simulink model "simulink_model"  (R2024b)
settings: Solver=FixedStepDiscrete  StartTime=0.0  StopTime=10.0  FixedStep=0.1  RelTol=1e-3  EnableMultiTasking=on
libraries: stm32f4xxblockslib x8, stm32blockslib x2
settings Model: STM32="{\"DigitalPortWrite\":[{\"ID\":\"untitled:4\"},{\"ID\":\"progetto:4\"},{\"ID\":\"progetto_gruppo17:4\"},{\"ID\":\"progetto_gruppo17:23\"},{\"ID\":\"progetto_gruppo17_05_06_2025:23\"},{\"ID\":\"progetto_gruppo17_05_06_2025:4\"},{\"ID\":\"progetto_gruppo17_06_06_2025:23\"},{\"ID\":\"progetto_gruppo17_06_06_2025:4\"},{\"ID\":\"progetto_gruppo17_06_06_2025_vers_a:4\"},{\"ID\":\"progetto_gruppo17_06_06_2025_vers_a:23\"},{\"ID\":\"progetto_se_gruppo_17:23\"},{\"ID\":\"progetto_se_gruppo_17:4\"}],\"DigitalPortRead\":[{\"ID\":\"untitled:5\"},{\"ID\":\"progetto:5\"},{\"ID\":\"progetto_gruppo17:5\"},{\"ID\":\"progetto_gruppo17:22\"},{\"ID\":\"progetto_gruppo17:24\"},{\"ID\":\"progetto_gruppo17:29\"},{\"ID\":\"progetto_gruppo17_05_06_2025:29\"},{\"ID\":\"progetto_gruppo17_05_06_2025:24\"},{\"ID\":\"progetto_gruppo17_05_06_2025:22\"},{\"ID\":\"progetto_gruppo17_05_06_2025:5\"},{\"ID\":\"progetto_gruppo17_06_06_2025:29\"},{\"ID\":\"progetto_gruppo17_06_06_2025:24\"},{\"ID\":\"progetto_gruppo17_06_06_2025:22\"},{\"ID\":\"progetto_gruppo17_06_06_2025:5\"},{\"ID\":\"progetto_gruppo17_06_06_2025_vers_a:5\"},{\"ID\":\"progetto_gruppo17_06_06_2025_vers_a:22\"},{\"ID\":\"progetto_gruppo17_06_06_2025_vers_a:24\"},{\"ID\":\"progetto_gruppo17_06_06_2025_vers_a:29\"},{\"ID\":\"progetto_se_gruppo_17:29\"},{\"ID\":\"progetto_se_gruppo_17:24\"},{\"ID\":\"progetto_se_gruppo_17:22\"},{\"ID\":\"progetto_se_gruppo_17:5\"}],\"UARTWrite\":[{\"ID\":\"untitled:10\"},{\"ID\":\"progetto:10\"},{\"ID\":\"progetto_gruppo17:10\"},{\"ID\":\"progetto_gruppo17_05_06_2025:10\"},{\"ID\":\"progetto_gruppo17_06_06_2025:10\"},{\"ID\":\"progetto_gruppo17_06_06_2025_vers_a:10\"},{\"ID\":\"progetto_se_gruppo_17:10\"}],\"UARTRead\":[{\"ID\":\"untitled:20\"},{\"ID\":\"progetto:20\"},{\"ID\":\"progetto_gruppo17:20\"},{\"ID\":\"progetto_gruppo17_05_06_2025:20\"},{\"ID\":\"progetto_gruppo17_06_06_2025:20\"},{\"ID\":\"progetto_gruppo17_06_06_2025_vers_a:20\"},{\"ID\":\"progetto_se_gruppo_17:20\"}],\"PWMOutput\":[{\"ID\":\"progetto_gruppo17:26\"},{\"ID\":\"progetto_gruppo17_05_06_2025:26\"},{\"ID\":\"progetto_gruppo17_05_06_2025:30\"},{\"ID\":\"progetto_gruppo17_06_06_2025:26\"},{\"ID\":\"progetto_gruppo17_06_06_2025:30\"},{\"ID\":\"progetto_gruppo17_06_06_2025_vers_a:30\"},{\"ID\":\"progetto_gruppo17_06_06_2025_vers_a:26\"},{\"ID\":\"progetto_se_gruppo_17:26\"},{\"ID\":\"progetto_se_gruppo_17:30\"}]}"  Creator=simon  LastModifiedBy=simon
settings OptimizationCC: DefaultParameterBehavior=Inlined  EnhancedBackFolding=on  PassReuseOutputArgsAs=Individual arguments  ZeroExternalMemoryAtStartup=off  ZeroInternalMemoryAtStartup=off  MaxStackSize=512  OptimizeBlockOrder=speed  DifferentSizesBufferReuse=on  OptimizationCustomize=off  EfficientTunableParamExpr=on
settings DebuggingCC: ParameterTunabilityLossMsg=error
settings HardwareCC: ProdBitPerPointer=32  ProdBitPerSizeT=32  ProdBitPerPtrDiffT=32  ProdLargestAtomicInteger=Long  ProdLargestAtomicFloat=Double  ProdWordSize=32  ProdLongLongMode=on  ProdHWDeviceType=ARM Compatible->ARM Cortex-M
settings SFSimCC: MATLABDynamicMemAlloc=off
settings RTWCC: Description=Embedded Coder  SystemTargetFile=ert.tlc  HardwareBoard=STM32G4xx Based  TemplateMakefile=ert_default_tmf  Toolchain=GNU Tools for ARM Embedded Processors
settings CodeAppCC: ForceParamTrailComments=on  IgnoreCustomStorageClasses=off  OperatorAnnotations=on  SimulinkDataObjDesc=on  SFDataObjDesc=on  InsertBlockDesc=on
settings ERTTargetCC: TargetLangStandard=C99 (ISO)  CodeReplacementLibrary=ARM Cortex-M  SupportVariableSizeSignals=on  ExtModeTransport=3  ExtModeStaticAlloc=on  ExtModeStaticAllocSize=2048  ExtModeMexFile=ext_xcp  ExtModeIntrfLevel=Level2 - Open  DynamicArrayContainerType=coder::array

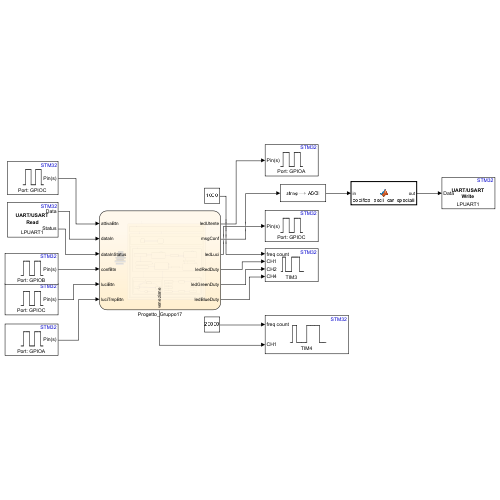
[thumbnail: Simulink's stored preview of the top-level diagram]
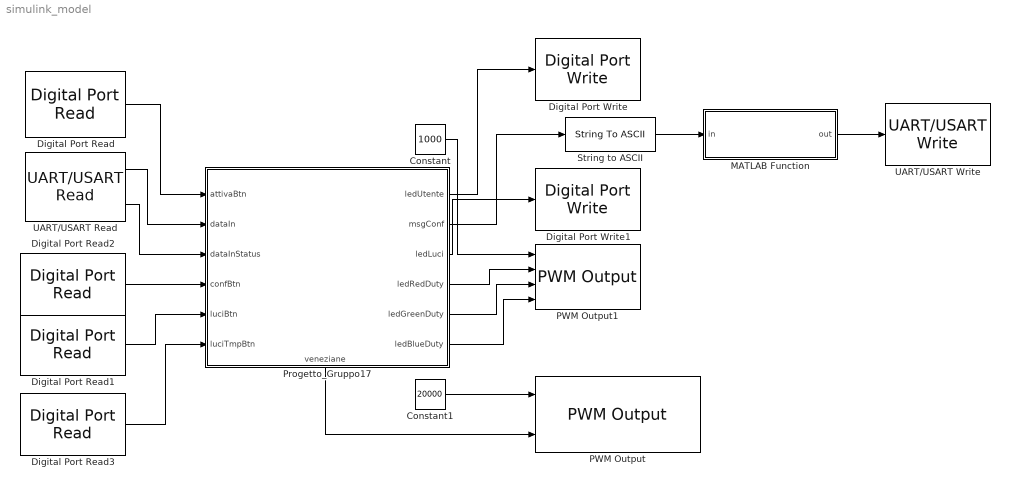
== system simulink_model ==
  Constant : Constant  Value=1000
  Constant1 : Constant  Value=20000
  Digital Port Read : stm32f4xxblockslib/Digital Port Read  PortName=GPIOC  PinNumber=[13]  ReadOperation=on  IOAsArray=on  SampleTime=-1  EnableSimPort=off  hoistedMaskSrc=ECSoC/ECSimCodegen/Digital Port Read
      settings: LibrarySourceBlock=stm32f2xxblockslib/Digital Port Read
  Digital Port Read1 : stm32f4xxblockslib/Digital Port Read  PortName=GPIOC  PinNumber=[10]  ReadOperation=on  IOAsArray=on  SampleTime=-1  EnableSimPort=off  hoistedMaskSrc=ECSoC/ECSimCodegen/Digital Port Read
      settings: LibrarySourceBlock=stm32f3xxblockslib/Digital Port Read
  Digital Port Read2 : stm32f4xxblockslib/Digital Port Read  PortName=GPIOB  PinNumber=[0]  ReadOperation=on  IOAsArray=on  SampleTime=-1  EnableSimPort=off  hoistedMaskSrc=ECSoC/ECSimCodegen/Digital Port Read
      settings: LibrarySourceBlock=stm32f3xxblockslib/Digital Port Read
  Digital Port Read3 : stm32f4xxblockslib/Digital Port Read  PortName=GPIOA  PinNumber=[15]  ReadOperation=on  IOAsArray=on  SampleTime=-1  EnableSimPort=off  hoistedMaskSrc=ECSoC/ECSimCodegen/Digital Port Read
      settings: LibrarySourceBlock=stm32f3xxblockslib/Digital Port Read
  Digital Port Write : stm32f4xxblockslib/Digital Port Write  PortName=GPIOA  PinNumber=[5]  ReadOperation=off  IOAsArray=on  EnableSimPort=off  hoistedMaskSrc=ECSoC/ECSimCodegen/Digital Port Write
      settings: LibrarySourceBlock=stm32f3xxblockslib/Digital Port Write
  Digital Port Write1 : stm32f4xxblockslib/Digital Port Write  PortName=GPIOC  PinNumber=[2]  ReadOperation=off  IOAsArray=on  EnableSimPort=off  hoistedMaskSrc=ECSoC/ECSimCodegen/Digital Port Write
      settings: LibrarySourceBlock=stm32f3xxblockslib/Digital Port Write
  MATLAB Function : MATLAB Function  TreatAsAtomicUnit=on
  PWM Output : stm32f4xxblockslib/PWM Output  TimerModule=TIM4  DutycycleUnits=Counts  EnableChannel1=on  EnableChannel2=off  EnableChannel3=off  EnableChannel4=off  EnableCounterInput=off  EnableMainOutputInput=off  EnableFrequencyInput=on  SetRCAfterCE=off  OutputDirection=off  OutputMainOutputEnableStatus=off  SampleTime=0.1  EnableSimPort=off  EnableUpdateEvent=off  EnableCaptureCompare1Event=off  EnableCaptureCompare2Event=off  EnableCaptureCompare3Event=off  EnableCaptureCompare4Event=off  EnableTriggerEvent=off  EnableBreakEvent=off  ProcessorFamily=STM32F4  hoistedMaskSrc=ECSoC/ECSimCodegen/PWM Output
      settings: LibrarySourceBlock=stm32f2xxblockslib/PWM Output
  PWM Output1 : stm32f4xxblockslib/PWM Output  TimerModule=TIM3  DutycycleUnits=Percentage  EnableChannel1=on  EnableChannel2=on  EnableChannel3=off  EnableChannel4=on  EnableCounterInput=off  EnableMainOutputInput=off  EnableFrequencyInput=on  SetRCAfterCE=off  OutputDirection=off  OutputMainOutputEnableStatus=off  SampleTime=0.1  EnableSimPort=off  EnableUpdateEvent=off  EnableCaptureCompare1Event=off  EnableCaptureCompare2Event=off  EnableCaptureCompare3Event=off  EnableCaptureCompare4Event=off  EnableTriggerEvent=off  EnableBreakEvent=off  ProcessorFamily=STM32F3  hoistedMaskSrc=ECSoC/ECSimCodegen/PWM Output
      settings: LibrarySourceBlock=stm32f3xxblockslib/PWM Output
  Progetto_Gruppo17 : Stateflow chart  TreatAsAtomicUnit=on
      settings: PortSchema="{\"entries\":[{\"content\":{\"sides\":[{\"content\":{\"connectorIds\":[\"In1\",\"In2\",\"In3\",\"In4\",\"In5\",\"In6\"]},\"type\":\"ConnectorPlacement.EquallySpacedRectSide\",\"uuid\":\"75f39260-4103-4749-81bf-ba76d3f8645b\"},{\"content\":{\"connectorIds\":[\"Out2\",\"Out3\",\"Out4\",\"Out7\",\"Out6\",\"Out5\"],\"side\":\"RIGHT\"},\"type\":\"ConnectorPlacement.EquallySpacedRectSide\",\"uuid\":\"22f09110-723e-4154-922d-9361e0bfb65a\"},{\"content\":{\"side\":\"TOP\"},\"type\":\"ConnectorPlacement.EquallySpacedRectSide\",\"uuid\":\"fa7b379e-0fd5-4b5f-9158-63c7f34f09a8\"},{\"content\":{\"connectorIds\":[\"Out1\"],\"side\":\"BOTTOM\"},\"type\":\"ConnectorPlacement.EquallySpacedRectSide\",\"uuid\":\"f8770b9f-bc27-4bf9-8903-206540cbe1f9\"}]},\"type\":\"ConnectorPlacement.EquallySpacedConnector\",\"uuid\":\"436e63a6-7db2-4b6a-ab66-b755d4d8d881\"}],\"packageUris\":[\"http://schema.mathworks.com/mf0/Connector/R2020b\"],\"version\":\"1.0\"}"
  String to ASCII : StringToASCII  OutputVectorSize=100
  UART/USART Read : stm32blockslib/UART//USART Read  UARTModule=LPUART1  DataType=uint8  DataLength=1  BlockingMode=off  BlockingTimeout=0.1  OutputLength=off  OutputStatus=on  SampleTime=-1
      settings: LibrarySourceBlock=stm32f2xxblockslib/UART//USART Read
  UART/USART Write : stm32blockslib/UART//USART Write  UARTModule=LPUART1  LengthOfDataToSend=off  BlockingMode=off  BlockingTimeout=0.1  OutputStatus=off
      settings: LibrarySourceBlock=stm32g4xxblockslib/UART//USART Write
  wires:
  Digital Port Read1/1 -> Progetto_Gruppo17/5(luciBtn)
  Digital Port Read3/1 -> Progetto_Gruppo17/6(luciTmpBtn)
  Constant/1 -> PWM Output1/1
  Digital Port Read/1 -> Progetto_Gruppo17/1(attivaBtn)
  Digital Port Read2/1 -> Progetto_Gruppo17/4(confBtn)
  UART/USART Read/2 -> Progetto_Gruppo17/3(dataInStatus)
  UART/USART Read/1 -> Progetto_Gruppo17/2(dataIn)
  Progetto_Gruppo17/1(veneziane) -> PWM Output/2
  Progetto_Gruppo17/6(ledGreenDuty) -> PWM Output1/3
  Progetto_Gruppo17/2(ledUtente) -> Digital Port Write/1
  Progetto_Gruppo17/7(ledRedDuty) -> PWM Output1/2
  Progetto_Gruppo17/3(msgConf) -> String to ASCII/1
  Progetto_Gruppo17/4(ledLuci) -> Digital Port Write1/1
  Progetto_Gruppo17/5(ledBlueDuty) -> PWM Output1/4
  Constant1/1 -> PWM Output/1
  String to ASCII/1 -> MATLAB Function/1(in)
  MATLAB Function/1(out) -> UART/USART Write/1

== stateflow chart simulink_model/Progetto_Gruppo17 ==
  state SistemaDomotica
    state SistemaInattivo
      en:attiva_btn_prev = attivaBtn;
      msgConf = "\033[0;0H\033[2JDISPOSITIVO INATTIVO :("
      ledUtente = OFF;
      ledLuci = OFF;
      ledBlueDuty = 100;
      ledGreenDuty = 0;
      ledRedDuty = 0;
      veneziane = dutyVeneziane(0);
      du: attiva_btn_prev = attivaBtn;
      msgConf = "";
    state SistemaAttivo
      en: attiva_btn_prev = attivaBtn;
      du: attiva_btn_prev = attivaBtn;
      state LedToggle [parallel]
        settings: executionOrder=1
        state LedOff
          en: ledUtente=OFF;
        state LedOn
          en: ledUtente=ON;
        (default) -> LedOn
        LedOn -> LedOff : after(0.5,sec)
        LedOff -> LedOn : after(0.5,sec)
      state ModSistema [parallel]
        settings: executionOrder=2
        state ConfigurazioneDispositivo
          en: conf_btn_prev = confBtn;
          du: conf_btn_prev = confBtn;
          state RicezioneStatoLuci
            en: valid=2; stato_luci = 2;
            if dataIn == char(13)
            [valid,stato_luci] = verificaValoreLuci(buffer);
            if stato_luci == TRUE && valid == TRUE
            msgConf = " -> ACCESE\n\r";
            elseif stato_luci == FALSE && valid == TRUE
            msgConf = " -> SPENTE\n\r";
            elseif valid == FALSE
            msgConf = "-> ERRORE\033[2K\r";
            end
            else
            [buffer, buffer_index, message] = gestisciBufferInput(dataIn, buffer, buffer_index,2);
            msgConf = string(char(message));
            end
            du:  msgConf = "";
          state RicezioneConfVeneziane
            en: valid = 2;
            if dataIn == char(13)
            gradi_veneziana_in = conversioneNum(buffer,buffer_index);
            valid = verificaValoreVeneziane(gradi_veneziana_in);
            if valid == TRUE
            msgConf = " -> OK\n\r";
            else
            msgConf = "-> ERRORE\033[2K\r";
            end
            buffer_index = 1;
            else
            [buffer, buffer_index, message] = gestisciBufferInput(dataIn, buffer, buffer_index,4);
            msgConf = string(char(message));
            end
            du:  msgConf = "";
          state StampaConfVeneziane
            en: msgConf="Configura veneziane - [0:180] (Gradi) - Risoluzione [20] (Gradi): ";
            buffer_index=1;
            du: msgConf="";
          state StampaConfStatoLuce
            en: msgConf="Configura luci - [a/A (Accese), s/S (Spente)]: ";
            buffer_index=1;
            du: msgConf="";
          state StampaConfTempLuce
            en: msgConf="Inserisci un valore di temporizzazione - [0] (Inattiva) - [5:30] (Secondi): ";
            buffer_index=1;
            du: msgConf="";
          state InizioConfigurazione
            en: conf_setted = FALSE;
            if valid_conf == TRUE
            msgConf = "\033[0;0H\033[2JMOD CONF [::]\n\r[EXIT MODE] Premi CONF_BTN per uscire...\n\r";
            else
            msgConf = "\033[0;0H\033[2JMOD CONF [::]\n\r";
            end
          state RicezioneTemperatura
            en: valid=2;
            if dataIn == char(13)
            temperatura = conversioneNum(buffer,buffer_index);
            valid = conversioneValoreTemperatura(temperatura);
            if valid == TRUE
            msgConf = " -> OK\n\r";
            else
            msgConf = "->ERRORE\033[2K\r";
            end
            buffer_index = 1;
            else
            [buffer, buffer_index, message] = gestisciBufferInput(dataIn, buffer, buffer_index,3);
            msgConf = string(char(message));
            end
            du:  msgConf = "";
          state RicezioneTempLuci
            en: valid=2;
            if dataIn == char(13)
            temporizzazione = conversioneNum(buffer,buffer_index);
            valid = conversioneValoreTemporizzazione(temporizzazione);
            if valid == TRUE
            msgConf = " -> OK\n\r";
            else
            msgConf = "-> ERRORE\033[2K\r";
            end
            buffer_index = 1;
            else
            [buffer, buffer_index, message] = gestisciBufferInput(dataIn, buffer, buffer_index,3);
            msgConf = string(char(message));
            end
            du:  msgConf = "";
          state FineConfigurazione
            en: conf_setted = TRUE; msgConf = "CONF DONE -> CONF EXIT\n"; valid_conf = TRUE;
            veneziane_conf_val = gradi_veneziana_in;
            stato_luci_conf_val = stato_luci;
            temp_luci_conf_val = temporizzazione;
            temperatura_conf_val = temperatura;
          state StampaConfTemperatura
            en: msgConf="Configura temperatura - [16:30] (Gradi): ";
            buffer_index=1;
            du: msgConf="";
          RicezioneStatoLuci -> RicezioneStatoLuci [order 1] : [dataInStatus==0]
          RicezioneConfVeneziane -> RicezioneConfVeneziane [order 1] : [dataInStatus==0]
          StampaConfVeneziane -> RicezioneConfVeneziane : [dataInStatus==0]
          StampaConfStatoLuce -> RicezioneStatoLuci : [dataInStatus==0]
          RicezioneConfVeneziane -> StampaConfStatoLuce [order 3] : [valid==TRUE]
          RicezioneConfVeneziane -> StampaConfVeneziane [order 2] : [valid==FALSE]
          RicezioneStatoLuci -> StampaConfStatoLuce [order 2] : [valid == FALSE]
          InizioConfigurazione -> StampaConfVeneziane : [conf_setted==FALSE]
          RicezioneStatoLuci -> StampaConfTempLuce [order 3] : [valid == TRUE]
          StampaConfTempLuce -> RicezioneTempLuci : [dataInStatus == 0]
          RicezioneTempLuci -> StampaConfTempLuce [order 2] : [valid == FALSE]
          RicezioneTempLuci -> RicezioneTempLuci [order 3] : [dataInStatus == 0]
          (default) -> InizioConfigurazione
          RicezioneTemperatura -> RicezioneTemperatura [order 2] : [dataInStatus == 0]
          RicezioneTemperatura -> FineConfigurazione [order 3] : [valid == TRUE]
          StampaConfTemperatura -> RicezioneTemperatura : [dataInStatus == 0]
          RicezioneTempLuci -> StampaConfTemperatura [order 1] : [valid == TRUE]
          RicezioneTemperatura -> StampaConfTemperatura [order 1] : [valid == FALSE]
        state EsecuzioneDispositivo
          en: conf_btn_prev = confBtn;
          msgConf = "\033[0;0H\033[2J";
          du: conf_btn_prev = confBtn;
          state StampaStato [parallel]
            settings: executionOrder=4
            state StatoVenezianeValue
              en: msgConf =string(veneziane_conf_val);
              du: msgConf = "";
            state StatoLuci
              if ledLuci == OFF
              msgConf = " gradi\n\rLuci: spente";
              else
              msgConf = " gradi\n\rLuci: accese";
              end
              du: msgConf = "";
            state StatoLuciTemporizzateDialog
              en: msgConf="\n\rDurata temporizzazione: "
              du: msgConf="";
            state StatoVenezianeDialog
              en: msgConf = "Veneziane: ";
              du: msgConf = "";
            state StatoLuciTemporizzateValue
              en: msgConf = string(temp_luci_conf_val);
              du: msgConf = "";
            state StatoOperativo
              msgConf = "\033[0;0H\033[2JMOD OPERATIVA ::>\n\r";
              du: msgConf = "";
            state StatoTemperaturaDialog
              en: msgConf = " sec\n\rTemperatura: ";
              du: msgConf= "";
            state StatoTemperaturaValue
              en: msgConf = string(temperatura_conf_val);
              du: msgConf= "";
            state StatoTemperaturaValue1
              en: msgConf = " gradi";
              du: msgConf= "";
            StatoVenezianeValue -> StatoLuci : [1]
            StatoLuci -> StatoLuciTemporizzateDialog : [1]
            StatoVenezianeDialog -> StatoVenezianeValue : [1]
            StatoLuciTemporizzateDialog -> StatoLuciTemporizzateValue : [1]
            StatoOperativo -> StatoVenezianeDialog : [1]
            (default) -> StatoOperativo
            StatoLuciTemporizzateValue -> StatoTemperaturaDialog : [1]
            StatoTemperaturaValue1 -> StatoOperativo : [after(10,sec)]
            StatoTemperaturaDialog -> StatoTemperaturaValue : [1]
            StatoTemperaturaValue -> StatoTemperaturaValue1 : [1]
          state GestoreTemperatura [parallel]
            en: [ledRedDuty, ledGreenDuty, ledBlueDuty]=cambioDuty(temperatura_conf_val);
            settings: executionOrder=1
          state GestoreVeneziane [parallel]
            en: veneziane = dutyVeneziane(veneziane_conf_val);
            settings: executionOrder=3
          state GestoreLuci [parallel]
            settings: executionOrder=2
            state AcceseTemp
              en:ledLuci = ON;
              luci_btn_prev = luciBtn;
              du: luci_btn_prev = luciBtn;
            state Spente
              en: ledLuci = OFF;
              luci_btn_prev = luciBtn;
              luci_temp_btn_prev = luciTmpBtn;
              du: luci_btn_prev = luciBtn;
              luci_temp_btn_prev = luciTmpBtn;
            state Accese
              en: ledLuci = ON;
              luci_btn_prev = luciBtn;
              luci_temp_btn_prev = luciTmpBtn;
              du: luci_btn_prev = luciBtn;
              luci_temp_btn_prev = luciTmpBtn;
            state StatoIniziale
              en: ledLuci = OFF;
            Spente -> AcceseTemp [order 2] : [temp_luci_conf_val ~= 0 && luci_temp_btn_prev == PRESSED && luciTmpBtn == NOTPRESSED]{luci_temp_btn_prev = luciTmpBtn;}
            Accese -> AcceseTemp [order 2] : [temp_luci_conf_val ~= 0 && luci_temp_btn_prev == PRESSED && luciTmpBtn == NOTPRESSED]{luci_temp_btn_prev = luciTmpBtn;}
            AcceseTemp -> Spente : [after(temp_luci_conf_val,sec) || (luci_btn_prev == PRESSED && luciBtn == NOTPRESSED)]{luci_btn_prev = luciBtn;}
            Accese -> Spente [order 1] : [luci_btn_prev == PRESSED && luciBtn == NOTPRESSED]{luci_btn_prev = luciBtn;}
            Spente -> Accese [order 1] : [luci_btn_prev == PRESSED && luciBtn == NOTPRESSED]{luci_btn_prev = luciBtn;}
            StatoIniziale -> Spente [order 1] : [stato_luci_conf_val == OFF]
            StatoIniziale -> Accese [order 2] : [stato_luci_conf_val == ON]
            (default) -> StatoIniziale
        (default) -> ConfigurazioneDispositivo
        ConfigurazioneDispositivo -> EsecuzioneDispositivo : [conf_setted == TRUE || (valid_conf == TRUE && confBtn == NOTPRESSED && conf_btn_prev == PRESSED)]{conf_btn_prev = confBtn;}
        EsecuzioneDispositivo -> ConfigurazioneDispositivo : [confBtn == NOTPRESSED && conf_btn_prev == PRESSED]{conf_btn_prev = confBtn;}
    (default) -> SistemaInattivo
    SistemaInattivo -> SistemaAttivo : [attivaBtn == NOTPRESSED && attiva_btn_prev == PRESSED]{attiva_btn_prev = attivaBtn}
    SistemaAttivo -> SistemaInattivo : [attivaBtn == NOTPRESSED && attiva_btn_prev == PRESSED]{attiva_btn_prev = attivaBtn;}
  (default) -> SistemaDomotica : {
      | attiva_btn_prev = NOTPRESSED;
      | conf_btn_prev = NOTPRESSED;
      | luci_btn_prev = NOTPRESSED;
      | luci_temp_btn_prev = NOTPRESSED;
      | conf_setted = FALSE;
      | }
  data: buff function_input; valido function_output; luci function_output; buff function_input; val function_output; buff_index function_input; valido function_output; gradi function_input; temp function_input; valido function_output; d function_input; buff function_input; buff_index function_input; buff function_output; buff_index function_output; msg function_output uint8; dimensione function_input; temp function_input; valido function_output; duty_red function_output; duty_green function_output; duty_blue function_output; temp function_input; gradi_ven function_input; impulso function_output; veneziane output =1; attivaBtn input; ledUtente output; msgConf output string =""; NOTPRESSED constant boolean =0; OFF constant double =0; ON constant double =1; PRESSED constant boolean =1; dataIn input uint8; dataInStatus input; buffer local uint8 size=6 =zeros(6,1); buffer_index local uint8; gradi_veneziana_in local uint8 =0; valid local uint8; message local uint8; stato_luci local uint8; temporizzazione local uint8; confBtn input; conf_setted local double =0; temperatura local uint8; luciBtn input; ledLuci output; stato_luci_conf_val local uint8 =0; temp_luci_conf_val local uint8 =0; temperatura_conf_val local uint8 =16; veneziane_conf_val local uint8 =0; valid_conf local double =0; ledBlueDuty output uint8 =100; ledGreenDuty output uint8 =0; ledRedDuty output uint8 =0; luciTmpBtn input; FALSE constant double =0; TRUE constant double =1; attiva_btn_prev local; conf_btn_prev local; luci_btn_prev local; luci_temp_btn_prev local
  function [valido,luci] = verificaValoreLuci(buff):
    | function [valido,luci] = verificaValoreLuci(buff)
    |     
    |     if buff(1) == char(65) || buff(1) == char(97)
    |          valido = uint8(1);
    |          luci = uint8(1);
    |     elseif buff(1) == char(83) || buff(1) == char(115)
    |          valido = uint8(1);
    |          luci = uint8(0);
    |     else
    |         valido = uint8(0);
    |         luci = uint8(2);
    |     end
    | 
    | end
  function val = conversioneNum(buff, buff_index):
    | function val = conversioneNum(buff, buff_index)
    | 
    |     val = uint8(0);
    |     j = uint8(1);
    | 
    |     while j < buff_index
    |         c = buff(j);
    |         if c >= uint8(48) && c <= uint8(57)
    |             val = val * uint8(10) + (c - uint8(48));
    |             j = j + 1;
    |         else
    |             val = uint8(255);  
    |             break;
    |         end
    |     end
    | end
  function valido = verificaValoreVeneziane(gradi):
    | function valido = verificaValoreVeneziane(gradi)
    |     if mod(gradi,20) == 0 && gradi >= 0 && gradi <= 180
    |         valido = uint8(1);
    |     else
    |         valido = uint8(0);
    |     end
    | end
  function valido = conversioneValoreTemporizzazione(temp):
    | function valido = conversioneValoreTemporizzazione(temp)
    |     if  temp >= 5 && temp <= 30 || temp == 0
    |         valido = uint8(1);
    |     else
    |         valido = uint8(0);
    |     end
    | end
  function [buff, buff_index,msg] = gestisciBufferInput(d, buff, buff_index,dimensione):
    | function [buff, buff_index,msg] = gestisciBufferInput(d, buff, buff_index,dimensione)
    |     
    |     msg = uint8(0);
    |     if  buff_index < dimensione && d ~= char(127)
    |         % Aggiunta normale di carattere
    |         buff(buff_index) = d;
    |         buff_index = buff_index + 1;
    |         msg = d;
    |     elseif d == char(127) && buff_index > 1
    |         % Backspace
    |         buff_index = buff_index - 1;
    |         msg = d;
    |     end
    | end
  function valido = conversioneValoreTemperatura(temp):
    | function valido = conversioneValoreTemperatura(temp)
    |     if  temp >= 16 && temp <= 30
    |         valido = uint8(1);
    |     else
    |         valido = uint8(0);
    |     end
    | end
  function [duty_red, duty_green, duty_blue] = cambioDuty(temp):
    | function [duty_red, duty_green, duty_blue] = cambioDuty(temp)
    | 
    | %blu
    | if temp >=16 && temp <=18
    |     duty_red = uint8(0);
    |     duty_green = uint8(0);
    |     duty_blue = uint8(100);
    | 
    | %viola
    | elseif temp >=19 && temp <=21
    |     duty_red = uint8(50);
    |     duty_green = uint8(0);
    |     duty_blue = uint8(50);
    | 
    | %giallo
    | elseif temp >= 22 && temp <=24
    |     duty_red = uint8(100);
    |     duty_green = uint8(10);
    |     duty_blue = uint8(0);
    | 
    | %arancione
    | elseif temp >= 25 && temp <= 27
    |     duty_red = uint8(100);
    |     duty_green = uint8(3);
    |     duty_blue = uint8(0);
    | 
    | %rosso
    | else
    |     duty_red = uint8(100);
    |     duty_green = uint8(0);
    |     duty_blue = uint8(0);
    | 
    | end
  function impulso = dutyVeneziane(gradi_ven):
    | function impulso = dutyVeneziane(gradi_ven)
    | 
    | gradi = double(gradi_ven);
    | impulso = 500 + (gradi *(2500 - 500) / 180);
    | 
    | end

== matlab function simulink_model/MATLAB Function ==
  data: in input; out output uint8 size=100
function out = codifica_ascii_car_speciali(in)

% Lunghezza massima supportata (personalizzabile)
MAX_LEN = 100;

% Preallocazione con lunghezza fissa
out = zeros(MAX_LEN,1, 'uint8');
len_out = 0;

i = 1;
while i <= length(in) && len_out < MAX_LEN
    
    if i + 15 <= length(in)
        if in(i)   == 92 && in(i+1) == 48 && in(i+2) == 51 && in(i+3) == 51 && ...
           in(i+4) == 91 && in(i+5) == 48 && in(i+6) == 59 && in(i+7) == 48 && ...
           in(i+8) == 72 && in(i+9) == 92 && in(i+10) == 48 && in(i+11) == 51 && ...
           in(i+12) == 51 && in(i+13) == 91 && in(i+14) == 50 && in(i+15) == 74
       
            if len_out + 10 <= MAX_LEN
                out(len_out+1:len_out+10) = uint8([27 91 48 59 48 72 27 91 50 74]);
                len_out = len_out + 10;
            end
            i = i + 16;
            continue;
        end
    end


    % Riconoscimento \033[2K = [92 48 51 51 91 50 75]
    if i + 6 <= length(in) && ...
       in(i)   == 92  && ...  % '\'
       in(i+1) == 48  && ...  % '0'
       in(i+2) == 51  && ...  % '3'
       in(i+3) == 51  && ...  % '3'
       in(i+4) == 91  && ...  % '['
       in(i+5) == 50  && ...  % '2'
       in(i+6) == 75          % 'K'
   
        % Sostituisci con [27 91 50 75]
        if len_out + 4 <= MAX_LEN
            out(len_out+1:len_out+4) = uint8([27 91 50 75]);
            len_out = len_out + 4;
        end
        i = i + 7;
        continue;
    end

    if in(i) == 92 && i < length(in)  % 92 == backslash '\'
        i = i + 1;
        if i <= length(in)
            c = in(i);
            esc_val = 0;
            switch c
                case 110  % 'n'
                    esc_val = 10;
                case 114  % 'r'
                    esc_val = 13;
                case 116  % 't'
                    esc_val = 9;
                case 92   % '\'
                    esc_val = 92;
                case 39   % '''
                    esc_val = 39;
                case 34   % '"'
                    esc_val = 34;
                otherwise
                    % Non riconosciuto, aggiungi '\' e il carattere successivo
                    len_out = len_out + 1;
                    out(len_out) = uint8(92);
                    if len_out < MAX_LEN
                        len_out = len_out + 1;
                        out(len_out) = uint8(c);
                    end
                    i = i + 1;
                    continue;
            end
            len_out = len_out + 1;
            out(len_out) = uint8(esc_val);
        end
    else
        len_out = len_out + 1;
        out(len_out) = uint8(in(i));
    end
    i = i + 1;
end
    
    disp(out)

end
